simulink model "controlVoltaje"  (R2020b)
settings: Solver=VariableStepAuto  StartTime=0.0  StopTime=10  RelTol=1e-3
libraries: powerlib x4
settings Model: Creator=petir  LastModifiedBy=petir

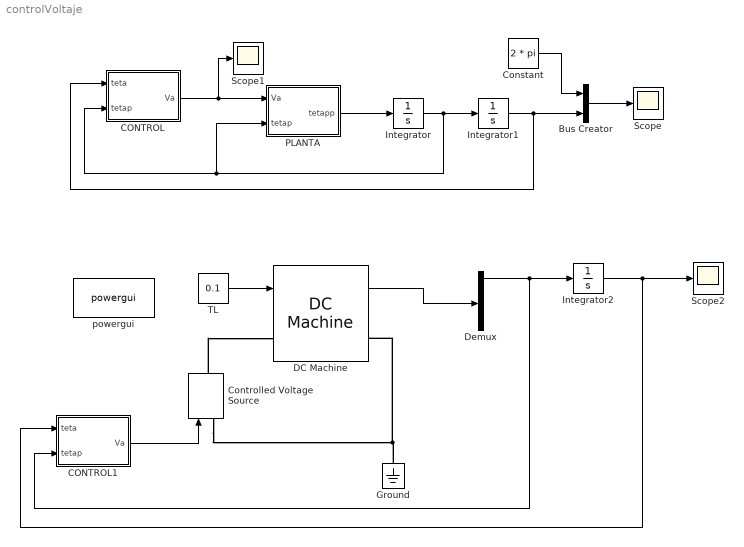
== system controlVoltaje ==
  Bus Creator : BusCreator  Inputs=2
  CONTROL : MATLAB Function  TreatAsAtomicUnit=on
  CONTROL1 : MATLAB Function  TreatAsAtomicUnit=on
  Constant : Constant  Value=2 * pi
  Controlled Voltage Source : powerlib/Electrical Sources/Controlled Voltage Source  Initialize=on  Source_Type=AC  Amplitude=0  Phase=0  Frequency=0  Measurements=None
  DC Machine : powerlib/Machines/DC Machine  PresetModel=No  MechanicalLoad=Torque TL  FieldType=Permanent magnet  ShowDetailedParameters=on  MeasurementBus=off  RLa=[ 8.3 1.51e-3]  RLf="[ 240  120]"  Laf=1.8  MachineConstant=Torque constant (N.m/A)  Ke=1.8  Kt=0.0879  J=80.7e-6  Bm=14.41e-6  Tf=0  w0=0  Ifinit=1  TsPowergui=0  TsBlock=-1
  Demux : Demux
  Ground : powerlib/Elements/Ground  LConnTagsString=a
  Integrator : Integrator
  Integrator1 : Integrator
  Integrator2 : Integrator
  PLANTA : MATLAB Function  TreatAsAtomicUnit=on
  Scope : Scope
  Scope1 : Scope
  Scope2 : Scope
  TL : Constant  Value=0.1
  powergui : powerlib/powergui  Priority=1  SimulationMode=Continuous  SampleTime=50e-6  frequency=60  Iterations=50  frequencyindice=0  Pbase=100e6  ErrMax=1e-4  UnitsV=kV  UnitsW=MW  buscounter=0  FunctionMessages=off  echomessages=off  EnableUseOfTLC=off  CurrentSourceSwitches=off  DisableSnubberDevices=off  DisableRonSwitches=off  DisableVfSwitches=off  DisplayEquations=off  AutomaticDiscreteSolvers=off  SolverType=Tustin/Backward Euler (TBE)  Interpol=off  ExternalGateDelay=off  methode=off  Ts=100  x0status=blocks  SPID=on  SwTol=0  HookPort=off  NonlinearTolerance=1e-4  nMaxIteration=100  ContinueOnMaxIteration=off  RestoreLinks=warning  ResistiveCurrentMeasurement=off  Frange=[0:2:500]  Ylog=off  Xlog=on  ShowGrid=off  save=off  variable=ZData  structure=0  ZoomFFT=off  StartTime=0.0  cycles=1  DisplayStyle=1  fundamental=60  FreqAxis=off  MaxFrequency=1000  frequencyindicesteady=1  RmsSteady=1  display=off
  wires:
  Integrator/1 -> CONTROL/2(tetap), PLANTA/2(tetap), Integrator1/1
  PLANTA/1(tetapp) -> Integrator/1
  CONTROL/1(Va) -> Scope1/1, PLANTA/1(Va)
  Bus Creator/1 -> Scope/1
  Integrator1/1 -> Bus Creator/2, CONTROL/1(teta)
  Constant/1 -> Bus Creator/1
  DC Machine/1 -> Demux/1
  TL/1 -> DC Machine/1
  Demux/1 -> CONTROL1/2(tetap), Integrator2/1
  CONTROL1/1(Va) -> Controlled Voltage Source/1
  Integrator2/1 -> CONTROL1/1(teta), Scope2/1
  connections:
  Controlled Voltage Source/RConn1 -- DC Machine/LConn1
  Controlled Voltage Source/LConn1 -- Ground/LConn1 -- DC Machine/RConn1

== matlab function controlVoltaje/PLANTA ==
  data: Va input; tetapp output; tetap input
function tetapp = fcn(Va, tetap)
% Parámetros
Ra = 8.3;
Ke = 0.0879;
Ki = 0.0879;
J = 80.7e-6;
B = 14.41e-6;
TL = 0.1;

tetapp = Ki / (J * Ra) * Va - Ki * Ke / (J * Ra) * tetap - B / J * tetap - 1 / J * TL;

== matlab function controlVoltaje/CONTROL1 ==
  data: teta input; Va output; tetap input
function Va = fcn(teta, tetap)
% Parametros
Ra = 8.3;
Ke = 0.0879;
Ki = 0.0879;
J = 80.7e-6;
B = 14.41e-6;
TL = 0.1;

tetad = 2 * pi;
Kp = 5;
Kd = 2;

Vaux = Kp * (tetad - teta) - Kd * tetap;
Va = J * Ra / Ki * (Vaux + Ki * Ke / (J * Ra) * tetap + B / J * tetap + 1 / J * TL);

== matlab function controlVoltaje/CONTROL ==
  data: teta input; Va output; tetap input
function Va = fcn(teta, tetap)
% Parametros
Ra = 8.3;
Ke = 0.0879;
Ki = 0.0879;
J = 80.7e-6;
B = 14.41e-6;
TL = 0.1;

tetad = 2 * pi;
Kp = 5;
Kd = 2;

Vaux = Kp * (tetad - teta) - Kd * tetap;
Va = J * Ra / Ki * (Vaux + Ki * Ke / (J * Ra) * tetap + B / J * tetap + 1 / J * TL);
